simulink model "Tilt_Controller"  (R2016a)
settings: Solver=VariableStepAuto  StartTime=0.0  StopTime=10  FixedStep=Ts  RelTol=1e-3
model workspace (MAT data in the model file):
  AC_ATTITUDE_ACCEL_Y_CONTROLLER_MAX_RADSS = Simulink.Signal
  AC_ATTITUDE_ACCEL_Y_CONTROLLER_MAX_RADSS.DataType = 'double'
  AC_ATTITUDE_ACCEL_Y_CONTROLLER_MAX_RADSS.Dimensions = 1
  AC_ATTITUDE_ACCEL_Y_CONTROLLER_MAX_RADSS.DimensionsMode = 'auto'
  AC_ATTITUDE_ACCEL_Y_CONTROLLER_MAX_RADSS.Complexity = 'real'
  AC_ATTITUDE_ACCEL_Y_CONTROLLER_MAX_RADSS.SampleTime = -1
  AC_ATTITUDE_ACCEL_Y_CONTROLLER_MAX_RADSS.SamplingMode = 'Sample based'
  AC_ATTITUDE_ACCEL_Y_CONTROLLER_MAX_RADSS.InitialValue = '0.5'
  AC_ATTITUDE_CONTROL_MAX = Simulink.Signal
  AC_ATTITUDE_CONTROL_MAX.DataType = 'double'
  AC_ATTITUDE_CONTROL_MAX.Dimensions = 1
  AC_ATTITUDE_CONTROL_MAX.DimensionsMode = 'auto'
  AC_ATTITUDE_CONTROL_MAX.Complexity = 'real'
  AC_ATTITUDE_CONTROL_MAX.SampleTime = -1
  AC_ATTITUDE_CONTROL_MAX.SamplingMode = 'Sample based'
  AC_ATTITUDE_CONTROL_MAX.InitialValue = '0.5'
  AC_ATTITUDE_THRUST_ERROR_ANGLE = Simulink.Signal
  AC_ATTITUDE_THRUST_ERROR_ANGLE.DataType = 'double'
  AC_ATTITUDE_THRUST_ERROR_ANGLE.Dimensions = 1
  AC_ATTITUDE_THRUST_ERROR_ANGLE.DimensionsMode = 'auto'
  AC_ATTITUDE_THRUST_ERROR_ANGLE.Complexity = 'real'
  AC_ATTITUDE_THRUST_ERROR_ANGLE.SampleTime = -1
  AC_ATTITUDE_THRUST_ERROR_ANGLE.SamplingMode = 'Sample based'
  AC_ATTITUDE_THRUST_ERROR_ANGLE.InitialValue = '1000'
  ROLL_PITCH_INPUT_MAX = Simulink.Signal
  ROLL_PITCH_INPUT_MAX.DataType = 'double'
  ROLL_PITCH_INPUT_MAX.Dimensions = 1
  ROLL_PITCH_INPUT_MAX.DimensionsMode = 'auto'
  ROLL_PITCH_INPUT_MAX.Complexity = 'real'
  ROLL_PITCH_INPUT_MAX.SampleTime = -1
  ROLL_PITCH_INPUT_MAX.SamplingMode = 'Sample based'
  ROLL_PITCH_INPUT_MAX.InitialValue = '3000'
  Sig = Simulink.Signal
  Sig.DataType = 'auto'
  Sig.Dimensions = -1
  Sig.DimensionsMode = 'auto'
  Sig.Complexity = 'auto'
  Sig.SampleTime = -1
  Sig.SamplingMode = 'auto'
  Sig1 = Simulink.Signal
  Sig1.DataType = 'auto'
  Sig1.Dimensions = -1
  Sig1.DimensionsMode = 'auto'
  Sig1.Complexity = 'auto'
  Sig1.SampleTime = -1
  Sig1.SamplingMode = 'auto'
  acro_yaw_p = Simulink.Signal
  acro_yaw_p.DataType = 'double'
  acro_yaw_p.Dimensions = 1
  acro_yaw_p.DimensionsMode = 'auto'
  acro_yaw_p.Complexity = 'real'
  acro_yaw_p.SampleTime = -1
  acro_yaw_p.SamplingMode = 'Sample based'
  acro_yaw_p.InitialValue = '45'
  angle_max = Simulink.Signal
  angle_max.DataType = 'double'
  angle_max.Dimensions = 1
  angle_max.DimensionsMode = 'auto'
  angle_max.Complexity = 'real'
  angle_max.SampleTime = -1
  angle_max.SamplingMode = 'Sample based'
  angle_max.InitialValue = '3000'
  attitude_target_ang_vel = Simulink.Signal
  attitude_target_ang_vel.DataType = 'double'
  attitude_target_ang_vel.Dimensions = 3
  attitude_target_ang_vel.DimensionsMode = 'auto'
  attitude_target_ang_vel.Complexity = 'real'
  attitude_target_ang_vel.SampleTime = -1
  attitude_target_ang_vel.SamplingMode = 'Sample based'
  attitude_target_ang_vel.InitialValue = '[0 0 0]'
  attitude_target_euler_angle_x = Simulink.Signal
  attitude_target_euler_angle_x.DataType = 'double'
  attitude_target_euler_angle_x.Dimensions = 1
  attitude_target_euler_angle_x.DimensionsMode = 'auto'
  attitude_target_euler_angle_x.Complexity = 'real'
  attitude_target_euler_angle_x.SampleTime = -1
  attitude_target_euler_angle_x.SamplingMode = 'Sample based'
  attitude_target_euler_angle_x.InitialValue = '0'
  attitude_target_euler_angle_y = Simulink.Signal
  attitude_target_euler_angle_y.DataType = 'double'
  attitude_target_euler_angle_y.Dimensions = 1
  attitude_target_euler_angle_y.DimensionsMode = 'auto'
  attitude_target_euler_angle_y.Complexity = 'real'
  attitude_target_euler_angle_y.SampleTime = -1
  attitude_target_euler_angle_y.SamplingMode = 'Sample based'
  attitude_target_euler_angle_y.InitialValue = '0'
  attitude_target_euler_angle_z = Simulink.Signal
  attitude_target_euler_angle_z.DataType = 'double'
  attitude_target_euler_angle_z.Dimensions = 1
  attitude_target_euler_angle_z.DimensionsMode = 'auto'
  attitude_target_euler_angle_z.Complexity = 'real'
  attitude_target_euler_angle_z.SampleTime = -1
  attitude_target_euler_angle_z.SamplingMode = 'Sample based'
  attitude_target_euler_angle_z.InitialValue = '0'
  attitude_target_euler_rate = Simulink.Signal
  attitude_target_euler_rate.DataType = 'double'
  attitude_target_euler_rate.Dimensions = 3
  attitude_target_euler_rate.DimensionsMode = 'auto'
  attitude_target_euler_rate.Complexity = 'real'
  attitude_target_euler_rate.SampleTime = -1
  attitude_target_euler_rate.SamplingMode = 'Sample based'
  attitude_target_euler_rate.InitialValue = '[0 0 0]'
  attitude_target_quat = Simulink.Signal
  attitude_target_quat.DataType = 'double'
  attitude_target_quat.Dimensions = 4
  attitude_target_quat.DimensionsMode = 'auto'
  attitude_target_quat.Complexity = 'real'
  attitude_target_quat.SampleTime = -1
  attitude_target_quat.SamplingMode = 'Sample based'
  attitude_target_quat.InitialValue = '[1 0 0 0]'
  attitude_vehicle_quat = Simulink.Signal
  attitude_vehicle_quat.DataType = 'double'
  attitude_vehicle_quat.Dimensions = 4
  attitude_vehicle_quat.DimensionsMode = 'auto'
  attitude_vehicle_quat.Complexity = 'real'
  attitude_vehicle_quat.SampleTime = -1
  attitude_vehicle_quat.SamplingMode = 'Sample based'
  attitude_vehicle_quat.InitialValue = '[1 0 0 0]'
  dt = Simulink.Signal
  dt.DataType = 'double'
  dt.Dimensions = 1
  dt.DimensionsMode = 'auto'
  dt.Complexity = 'real'
  dt.SampleTime = -1
  dt.SamplingMode = 'Sample based'
  dt.InitialValue = '0.01'
  false = 0
  limit_roll_pitch = Simulink.Signal
  limit_roll_pitch.DataType = 'double'
  limit_roll_pitch.Dimensions = 1
  limit_roll_pitch.DimensionsMode = 'auto'
  limit_roll_pitch.Complexity = 'real'
  limit_roll_pitch.SampleTime = -1
  limit_roll_pitch.SamplingMode = 'Sample based'
  limit_roll_pitch.InitialValue = '0.0'
  limit_throttle_upper = Simulink.Signal
  limit_throttle_upper.DataType = 'logical'
  limit_throttle_upper.Dimensions = 1
  limit_throttle_upper.DimensionsMode = 'auto'
  limit_throttle_upper.Complexity = 'real'
  limit_throttle_upper.SampleTime = -1
  limit_throttle_upper.SamplingMode = 'Sample based'
  limit_throttle_upper.InitialValue = '0'
  limit_yaw = Simulink.Signal
  limit_yaw.DataType = 'double'
  limit_yaw.Dimensions = 1
  limit_yaw.DimensionsMode = 'auto'
  limit_yaw.Complexity = 'real'
  limit_yaw.SampleTime = -1
  limit_yaw.SamplingMode = 'Sample based'
  limit_yaw.InitialValue = '0'
  loop_rate = Simulink.Signal
  loop_rate.DataType = 'double'
  loop_rate.Dimensions = 1
  loop_rate.DimensionsMode = 'auto'
  loop_rate.Complexity = 'real'
  loop_rate.SampleTime = -1
  loop_rate.SamplingMode = 'Sample based'
  loop_rate.InitialValue = '100'
  pitch_attitude_kP = Simulink.Signal
  pitch_attitude_kP.DataType = 'double'
  pitch_attitude_kP.Dimensions = 1
  pitch_attitude_kP.DimensionsMode = 'auto'
  pitch_attitude_kP.Complexity = 'real'
  pitch_attitude_kP.SampleTime = -1
  pitch_attitude_kP.SamplingMode = 'Sample based'
  pitch_attitude_kP.InitialValue = '20'
  pitch_factor = Simulink.Signal
  pitch_factor.DataType = 'double'
  pitch_factor.Dimensions = 4
  pitch_factor.DimensionsMode = 'auto'
  pitch_factor.Complexity = 'real'
  pitch_factor.SampleTime = -1
  pitch_factor.SamplingMode = 'Sample based'
  pitch_factor.InitialValue = '[cos(deg2rad(15)) -cos(deg2rad(15)) cos(deg2rad(15)) -cos(deg2rad(15))]'
  pitch_rate_derivative = Simulink.Signal
  pitch_rate_derivative.DataType = 'double'
  pitch_rate_derivative.Dimensions = 1
  pitch_rate_derivative.DimensionsMode = 'auto'
  pitch_rate_derivative.Complexity = 'real'
  pitch_rate_derivative.SampleTime = -1
  pitch_rate_derivative.SamplingMode = 'Sample based'
  pitch_rate_derivative.InitialValue = '0'
  pitch_rate_error_rads = Simulink.Signal
  pitch_rate_error_rads.DataType = 'double'
  pitch_rate_error_rads.Dimensions = 1
  pitch_rate_error_rads.DimensionsMode = 'auto'
  pitch_rate_error_rads.Complexity = 'real'
  pitch_rate_error_rads.SampleTime = -1
  pitch_rate_error_rads.SamplingMode = 'Sample based'
  pitch_rate_error_rads.InitialValue = '0'
  pitch_rate_filt_hz = Simulink.Signal
  pitch_rate_filt_hz.DataType = 'double'
  pitch_rate_filt_hz.Dimensions = 1
  pitch_rate_filt_hz.DimensionsMode = 'auto'
  pitch_rate_filt_hz.Complexity = 'real'
  pitch_rate_filt_hz.SampleTime = -1
  pitch_rate_filt_hz.SamplingMode = 'Sample based'
  pitch_rate_filt_hz.InitialValue = '1/(2*pi)'
  pitch_rate_imax = Simulink.Signal
  pitch_rate_imax.DataType = 'double'
  pitch_rate_imax.Dimensions = 1
  pitch_rate_imax.DimensionsMode = 'auto'
  pitch_rate_imax.Complexity = 'real'
  pitch_rate_imax.SampleTime = -1
  pitch_rate_imax.SamplingMode = 'Sample based'
  pitch_rate_imax.InitialValue = '200'
  pitch_rate_integrator = Simulink.Signal
  pitch_rate_integrator.DataType = 'double'
  pitch_rate_integrator.Dimensions = 1
  pitch_rate_integrator.DimensionsMode = 'auto'
  pitch_rate_integrator.Complexity = 'real'
  pitch_rate_integrator.SampleTime = -1
  pitch_rate_integrator.SamplingMode = 'Sample based'
  pitch_rate_integrator.InitialValue = '0'
  pitch_rate_kD = Simulink.Signal
  pitch_rate_kD.DataType = 'double'
  pitch_rate_kD.Dimensions = 1
  pitch_rate_kD.DimensionsMode = 'auto'
  pitch_rate_kD.Complexity = 'real'
  pitch_rate_kD.SampleTime = -1
  pitch_rate_kD.SamplingMode = 'Sample based'
  pitch_rate_kD.InitialValue = '0.004'
  pitch_rate_kI = Simulink.Signal
  pitch_rate_kI.DataType = 'double'
  pitch_rate_kI.Dimensions = 1
  pitch_rate_kI.DimensionsMode = 'auto'
  pitch_rate_kI.Complexity = 'real'
  pitch_rate_kI.SampleTime = -1
  pitch_rate_kI.SamplingMode = 'Sample based'
  pitch_rate_kI.InitialValue = '0.1'
  pitch_rate_kP = Simulink.Signal
  pitch_rate_kP.DataType = 'double'
  pitch_rate_kP.Dimensions = 1
  pitch_rate_kP.DimensionsMode = 'auto'
  pitch_rate_kP.Complexity = 'real'
  pitch_rate_kP.SampleTime = -1
  pitch_rate_kP.SamplingMode = 'Sample based'
  pitch_rate_kP.InitialValue = '0.5'
  pitch_rate_last_input = Simulink.Signal
  pitch_rate_last_input.DataType = 'double'
  pitch_rate_last_input.Dimensions = 1
  pitch_rate_last_input.DimensionsMode = 'auto'
  pitch_rate_last_input.Complexity = 'real'
  pitch_rate_last_input.SampleTime = -1
  pitch_rate_last_input.SamplingMode = 'Sample based'
  pitch_rate_last_input.InitialValue = '0'
  pitch_rate_proportional = Simulink.Signal
  pitch_rate_proportional.DataType = 'double'
  pitch_rate_proportional.Dimensions = 1
  pitch_rate_proportional.DimensionsMode = 'auto'
  pitch_rate_proportional.Complexity = 'real'
  pitch_rate_proportional.SampleTime = -1
  pitch_rate_proportional.SamplingMode = 'Sample based'
  pitch_rate_proportional.InitialValue = '0'
  pwm_max = Simulink.Signal
  pwm_max.DataType = 'double'
  pwm_max.Dimensions = 1
  pwm_max.DimensionsMode = 'auto'
  pwm_max.Complexity = 'real'
  pwm_max.SampleTime = -1
  pwm_max.SamplingMode = 'Sample based'
  pwm_max.InitialValue = '2000'
  pwm_min = Simulink.Signal
  pwm_min.DataType = 'double'
  pwm_min.Dimensions = 1
  pwm_min.DimensionsMode = 'auto'
  pwm_min.Complexity = 'real'
  pwm_min.SampleTime = -1
  pwm_min.SamplingMode = 'Sample based'
  pwm_min.InitialValue = '1039'
  rate_bf_ff_enabled = Simulink.Signal
  rate_bf_ff_enabled.DataType = 'double'
  rate_bf_ff_enabled.Dimensions = 1
  rate_bf_ff_enabled.DimensionsMode = 'auto'
  rate_bf_ff_enabled.Complexity = 'real'
  rate_bf_ff_enabled.SampleTime = -1
  rate_bf_ff_enabled.SamplingMode = 'Sample based'
  rate_bf_ff_enabled.InitialValue = '0'
  rate_target_ang_vel = Simulink.Signal
  rate_target_ang_vel.DataType = 'double'
  rate_target_ang_vel.Dimensions = 3
  rate_target_ang_vel.DimensionsMode = 'auto'
  rate_target_ang_vel.Complexity = 'real'
  rate_target_ang_vel.SampleTime = -1
  rate_target_ang_vel.SamplingMode = 'Sample based'
  rate_target_ang_vel.InitialValue = '[0 0 0]'
  roll_attitude_kP = Simulink.Signal
  roll_attitude_kP.DataType = 'double'
  roll_attitude_kP.Dimensions = 1
  roll_attitude_kP.DimensionsMode = 'auto'
  roll_attitude_kP.Complexity = 'real'
  roll_attitude_kP.SampleTime = -1
  roll_attitude_kP.SamplingMode = 'Sample based'
  roll_attitude_kP.InitialValue = '20'
  roll_factor = Simulink.Signal
  roll_factor.DataType = 'double'
  roll_factor.Dimensions = 4
  roll_factor.DimensionsMode = 'auto'
  roll_factor.Complexity = 'real'
  roll_factor.SampleTime = -1
  roll_factor.SamplingMode = 'Sample based'
  roll_factor.InitialValue = '[-sin(deg2rad(15)) sin(deg2rad(15)) sin(deg2rad(15)) -sin(deg2rad(15))]'
  roll_rate_derivative = Simulink.Signal
  roll_rate_derivative.DataType = 'double'
  roll_rate_derivative.Dimensions = 1
  roll_rate_derivative.DimensionsMode = 'auto'
  roll_rate_derivative.Complexity = 'real'
  roll_rate_derivative.SampleTime = -1
  roll_rate_derivative.SamplingMode = 'Sample based'
  roll_rate_derivative.InitialValue = '0'
  roll_rate_error_rads = Simulink.Signal
  roll_rate_error_rads.DataType = 'double'
  roll_rate_error_rads.Dimensions = 1
  roll_rate_error_rads.DimensionsMode = 'auto'
  roll_rate_error_rads.Complexity = 'real'
  roll_rate_error_rads.SampleTime = -1
  roll_rate_error_rads.SamplingMode = 'Sample based'
  roll_rate_error_rads.InitialValue = '0'
  roll_rate_filt_hz = Simulink.Signal
  roll_rate_filt_hz.DataType = 'double'
  roll_rate_filt_hz.Dimensions = 1
  roll_rate_filt_hz.DimensionsMode = 'auto'
  roll_rate_filt_hz.Complexity = 'real'
  roll_rate_filt_hz.SampleTime = -1
  roll_rate_filt_hz.SamplingMode = 'Sample based'
  roll_rate_filt_hz.InitialValue = '1/(2*pi)'
  roll_rate_imax = Simulink.Signal
  roll_rate_imax.DataType = 'double'
  roll_rate_imax.Dimensions = 1
  roll_rate_imax.DimensionsMode = 'auto'
  roll_rate_imax.Complexity = 'real'
  roll_rate_imax.SampleTime = -1
  roll_rate_imax.SamplingMode = 'Sample based'
  roll_rate_imax.InitialValue = '200'
  roll_rate_integrator = Simulink.Signal
  roll_rate_integrator.DataType = 'double'
  roll_rate_integrator.Dimensions = 1
  roll_rate_integrator.DimensionsMode = 'auto'
  roll_rate_integrator.Complexity = 'real'
  roll_rate_integrator.SampleTime = -1
  roll_rate_integrator.SamplingMode = 'Sample based'
  roll_rate_integrator.InitialValue = '0'
  roll_rate_kD = Simulink.Signal
  roll_rate_kD.DataType = 'double'
  roll_rate_kD.Dimensions = 1
  roll_rate_kD.DimensionsMode = 'auto'
  roll_rate_kD.Complexity = 'real'
  roll_rate_kD.SampleTime = -1
  roll_rate_kD.SamplingMode = 'Sample based'
  roll_rate_kD.InitialValue = '0.004'
  roll_rate_kI = Simulink.Signal
  roll_rate_kI.DataType = 'double'
  roll_rate_kI.Dimensions = 1
  roll_rate_kI.DimensionsMode = 'auto'
  roll_rate_kI.Complexity = 'real'
  roll_rate_kI.SampleTime = -1
  roll_rate_kI.SamplingMode = 'Sample based'
  roll_rate_kI.InitialValue = '0.1'
  roll_rate_kP = Simulink.Signal
  roll_rate_kP.DataType = 'double'
  roll_rate_kP.Dimensions = 1
  roll_rate_kP.DimensionsMode = 'auto'
  roll_rate_kP.Complexity = 'real'
  roll_rate_kP.SampleTime = -1
  roll_rate_kP.SamplingMode = 'Sample based'
  roll_rate_kP.InitialValue = '1'
  roll_rate_last_input = Simulink.Signal
  roll_rate_last_input.DataType = 'double'
  roll_rate_last_input.Dimensions = 1
  roll_rate_last_input.DimensionsMode = 'auto'
  roll_rate_last_input.Complexity = 'real'
  roll_rate_last_input.SampleTime = -1
  roll_rate_last_input.SamplingMode = 'Sample based'
  roll_rate_last_input.InitialValue = '0'
  roll_rate_proportional = Simulink.Signal
  roll_rate_proportional.DataType = 'double'
  roll_rate_proportional.Dimensions = 1
  roll_rate_proportional.DimensionsMode = 'auto'
  roll_rate_proportional.Complexity = 'real'
  roll_rate_proportional.SampleTime = -1
  roll_rate_proportional.SamplingMode = 'Sample based'
  roll_rate_proportional.InitialValue = '0'
  spin_max = Simulink.Signal
  spin_max.DataType = 'double'
  spin_max.Dimensions = 1
  spin_max.DimensionsMode = 'auto'
  spin_max.Complexity = 'real'
  spin_max.SampleTime = -1
  spin_max.SamplingMode = 'Sample based'
  spin_max.InitialValue = '0.95'
  spin_min = Simulink.Signal
  spin_min.DataType = 'double'
  spin_min.Dimensions = 1
  spin_min.DimensionsMode = 'auto'
  spin_min.Complexity = 'real'
  spin_min.SampleTime = -1
  spin_min.SamplingMode = 'Sample based'
  spin_min.InitialValue = '0.15'
  throttle_avg_max = Simulink.Signal
  throttle_avg_max.DataType = 'double'
  throttle_avg_max.Dimensions = 1
  throttle_avg_max.DimensionsMode = 'auto'
  throttle_avg_max.Complexity = 'real'
  throttle_avg_max.SampleTime = -1
  throttle_avg_max.SamplingMode = 'Sample based'
  throttle_avg_max.InitialValue = '0'
  throttle_filter_cutoff_freq = Simulink.Signal
  throttle_filter_cutoff_freq.DataType = 'double'
  throttle_filter_cutoff_freq.Dimensions = 1
  throttle_filter_cutoff_freq.DimensionsMode = 'auto'
  throttle_filter_cutoff_freq.Complexity = 'real'
  throttle_filter_cutoff_freq.SampleTime = -1
  throttle_filter_cutoff_freq.SamplingMode = 'Sample based'
  throttle_filter_cutoff_freq.InitialValue = '0.5'
  throttle_filter_output = Simulink.Signal
  throttle_filter_output.DataType = 'double'
  throttle_filter_output.Dimensions = 1
  throttle_filter_output.DimensionsMode = 'auto'
  throttle_filter_output.Complexity = 'real'
  throttle_filter_output.SampleTime = -1
  throttle_filter_output.SamplingMode = 'Sample based'
  throttle_filter_output.InitialValue = '0'
  throttle_in = Simulink.Signal
  throttle_in.DataType = 'double'
  throttle_in.Dimensions = 1
  throttle_in.DimensionsMode = 'auto'
  throttle_in.Complexity = 'real'
  throttle_in.SampleTime = -1
  throttle_in.SamplingMode = 'Sample based'
  throttle_in.InitialValue = '0'
  throttle_rpy_mix = Simulink.Signal
  throttle_rpy_mix.DataType = 'double'
  throttle_rpy_mix.Dimensions = 1
  throttle_rpy_mix.DimensionsMode = 'auto'
  throttle_rpy_mix.Complexity = 'real'
  throttle_rpy_mix.SampleTime = -1
  throttle_rpy_mix.SamplingMode = 'Sample based'
  throttle_rpy_mix.InitialValue = '0'
  throttle_rpy_mix_desired = Simulink.Signal
  throttle_rpy_mix_desired.DataType = 'double'
  throttle_rpy_mix_desired.Dimensions = 1
  throttle_rpy_mix_desired.DimensionsMode = 'auto'
  throttle_rpy_mix_desired.Complexity = 'real'
  throttle_rpy_mix_desired.SampleTime = -1
  throttle_rpy_mix_desired.SamplingMode = 'Sample based'
  throttle_rpy_mix_desired.InitialValue = '0'
  throttle_thrust = Simulink.Signal
  throttle_thrust.DataType = 'double'
  throttle_thrust.Dimensions = 1
  throttle_thrust.DimensionsMode = 'auto'
  throttle_thrust.Complexity = 'real'
  throttle_thrust.SampleTime = -1
  throttle_thrust.SamplingMode = 'Sample based'
  throttle_thrust.InitialValue = '0'
  throttle_thrust_best_rpy = Simulink.Signal
  throttle_thrust_best_rpy.DataType = 'double'
  throttle_thrust_best_rpy.Dimensions = 1
  throttle_thrust_best_rpy.DimensionsMode = 'auto'
  throttle_thrust_best_rpy.Complexity = 'real'
  throttle_thrust_best_rpy.SampleTime = -1
  throttle_thrust_best_rpy.SamplingMode = 'Sample based'
  throttle_thrust_best_rpy.InitialValue = '0'
  throttle_thrust_max = Simulink.Signal
  throttle_thrust_max.DataType = 'double'
  throttle_thrust_max.Dimensions = 1
  throttle_thrust_max.DimensionsMode = 'auto'
  throttle_thrust_max.Complexity = 'real'
  throttle_thrust_max.SampleTime = -1
  throttle_thrust_max.SamplingMode = 'Sample based'
  throttle_thrust_max.InitialValue = '1'
  thrust_error_angle = Simulink.Signal
  thrust_error_angle.DataType = 'double'
  thrust_error_angle.Dimensions = 1
  thrust_error_angle.DimensionsMode = 'auto'
  thrust_error_angle.Complexity = 'real'
  thrust_error_angle.SampleTime = -1
  thrust_error_angle.SamplingMode = 'Sample based'
  thrust_error_angle.InitialValue = '0'
  thrust_rpyt_out = Simulink.Signal
  thrust_rpyt_out.DataType = 'double'
  thrust_rpyt_out.Dimensions = 4
  thrust_rpyt_out.DimensionsMode = 'auto'
  thrust_rpyt_out.Complexity = 'real'
  thrust_rpyt_out.SampleTime = -1
  thrust_rpyt_out.SamplingMode = 'Sample based'
  thrust_rpyt_out.InitialValue = '[0 0 0 0]'
  true = 1
  use_ff_and_input_shaping = Simulink.Signal
  use_ff_and_input_shaping.DataType = 'double'
  use_ff_and_input_shaping.Dimensions = 1
  use_ff_and_input_shaping.DimensionsMode = 'auto'
  use_ff_and_input_shaping.Complexity = 'real'
  use_ff_and_input_shaping.SampleTime = -1
  use_ff_and_input_shaping.SamplingMode = 'Sample based'
  use_ff_and_input_shaping.InitialValue = '0'
  variableType = 'S'
  yaw_allowed = Simulink.Signal
  yaw_allowed.DataType = 'double'
  yaw_allowed.Dimensions = 1
  yaw_allowed.DimensionsMode = 'auto'
  yaw_allowed.Complexity = 'real'
  yaw_allowed.SampleTime = -1
  yaw_allowed.SamplingMode = 'Sample based'
  yaw_allowed.InitialValue = '1'
  yaw_attitude_kP = Simulink.Signal
  yaw_attitude_kP.DataType = 'double'
  yaw_attitude_kP.Dimensions = 1
  yaw_attitude_kP.DimensionsMode = 'auto'
  yaw_attitude_kP.Complexity = 'real'
  yaw_attitude_kP.SampleTime = -1
  yaw_attitude_kP.SamplingMode = 'Sample based'
  yaw_attitude_kP.InitialValue = '4.5'
  yaw_factor = Simulink.Signal
  yaw_factor.DataType = 'double'
  yaw_factor.Dimensions = 4
  yaw_factor.DimensionsMode = 'auto'
  yaw_factor.Complexity = 'real'
  yaw_factor.SampleTime = -1
  yaw_factor.SamplingMode = 'Sample based'
  yaw_factor.InitialValue = '[0.1 0.1 -0.1 -0.1]'
  yaw_headroom = Simulink.Signal
  yaw_headroom.DataType = 'double'
  yaw_headroom.Dimensions = 1
  yaw_headroom.DimensionsMode = 'auto'
  yaw_headroom.Complexity = 'real'
  yaw_headroom.SampleTime = -1
  yaw_headroom.SamplingMode = 'Sample based'
  yaw_headroom.InitialValue = '200'
  yaw_rate_derivative = Simulink.Signal
  yaw_rate_derivative.DataType = 'double'
  yaw_rate_derivative.Dimensions = 1
  yaw_rate_derivative.DimensionsMode = 'auto'
  yaw_rate_derivative.Complexity = 'real'
  yaw_rate_derivative.SampleTime = -1
  yaw_rate_derivative.SamplingMode = 'Sample based'
  yaw_rate_derivative.InitialValue = '0'
  yaw_rate_error_rads = Simulink.Signal
  yaw_rate_error_rads.DataType = 'double'
  yaw_rate_error_rads.Dimensions = 1
  yaw_rate_error_rads.DimensionsMode = 'auto'
  yaw_rate_error_rads.Complexity = 'real'
  yaw_rate_error_rads.SampleTime = -1
  yaw_rate_error_rads.SamplingMode = 'Sample based'
  yaw_rate_error_rads.InitialValue = '0'
  yaw_rate_filt_hz = Simulink.Signal
  yaw_rate_filt_hz.DataType = 'double'
  yaw_rate_filt_hz.Dimensions = 1
  yaw_rate_filt_hz.DimensionsMode = 'auto'
  yaw_rate_filt_hz.Complexity = 'real'
  yaw_rate_filt_hz.SampleTime = -1
  yaw_rate_filt_hz.SamplingMode = 'Sample based'
  yaw_rate_filt_hz.InitialValue = '1/(2*pi)'
  yaw_rate_imax = Simulink.Signal
  yaw_rate_imax.DataType = 'double'
  yaw_rate_imax.Dimensions = 1
  yaw_rate_imax.DimensionsMode = 'auto'
  yaw_rate_imax.Complexity = 'real'
  yaw_rate_imax.SampleTime = -1
  yaw_rate_imax.SamplingMode = 'Sample based'
  yaw_rate_imax.InitialValue = '200'
  yaw_rate_integrator = Simulink.Signal
  yaw_rate_integrator.DataType = 'double'
  yaw_rate_integrator.Dimensions = 1
  yaw_rate_integrator.DimensionsMode = 'auto'
  yaw_rate_integrator.Complexity = 'real'
  yaw_rate_integrator.SampleTime = -1
  yaw_rate_integrator.SamplingMode = 'Sample based'
  yaw_rate_integrator.InitialValue = '0'
  yaw_rate_kD = Simulink.Signal
  yaw_rate_kD.DataType = 'double'
  yaw_rate_kD.Dimensions = 1
  yaw_rate_kD.DimensionsMode = 'auto'
  yaw_rate_kD.Complexity = 'real'
  yaw_rate_kD.SampleTime = -1
  yaw_rate_kD.SamplingMode = 'Sample based'
  yaw_rate_kD.InitialValue = '5'
  yaw_rate_kI = Simulink.Signal
  yaw_rate_kI.DataType = 'double'
  yaw_rate_kI.Dimensions = 1
  yaw_rate_kI.DimensionsMode = 'auto'
  yaw_rate_kI.Complexity = 'real'
  yaw_rate_kI.SampleTime = -1
  yaw_rate_kI.SamplingMode = 'Sample based'
  yaw_rate_kI.InitialValue = '0.1'
  yaw_rate_kP = Simulink.Signal
  yaw_rate_kP.DataType = 'double'
  yaw_rate_kP.Dimensions = 1
  yaw_rate_kP.DimensionsMode = 'auto'
  yaw_rate_kP.Complexity = 'real'
  yaw_rate_kP.SampleTime = -1
  yaw_rate_kP.SamplingMode = 'Sample based'
  yaw_rate_kP.InitialValue = '0.2'
  yaw_rate_last_input = Simulink.Signal
  yaw_rate_last_input.DataType = 'double'
  yaw_rate_last_input.Dimensions = 1
  yaw_rate_last_input.DimensionsMode = 'auto'
  yaw_rate_last_input.Complexity = 'real'
  yaw_rate_last_input.SampleTime = -1
  yaw_rate_last_input.SamplingMode = 'Sample based'
  yaw_rate_last_input.InitialValue = '0'
  yaw_rate_proportional = Simulink.Signal
  yaw_rate_proportional.DataType = 'double'
  yaw_rate_proportional.Dimensions = 1
  yaw_rate_proportional.DimensionsMode = 'auto'
  yaw_rate_proportional.Complexity = 'real'
  yaw_rate_proportional.SampleTime = -1
  yaw_rate_proportional.SamplingMode = 'Sample based'
  yaw_rate_proportional.InitialValue = '0'
libraries: simulink_extras x6, vrlib x2, aerolibtransform2 x2, aerolibutil x1
settings Model: Creator=s121814  LastModifiedBy=GusBus
settings SolverCC: ZeroCrossControl=DisableAll
settings DataIOCC: SaveFormat=Array  SaveState=on

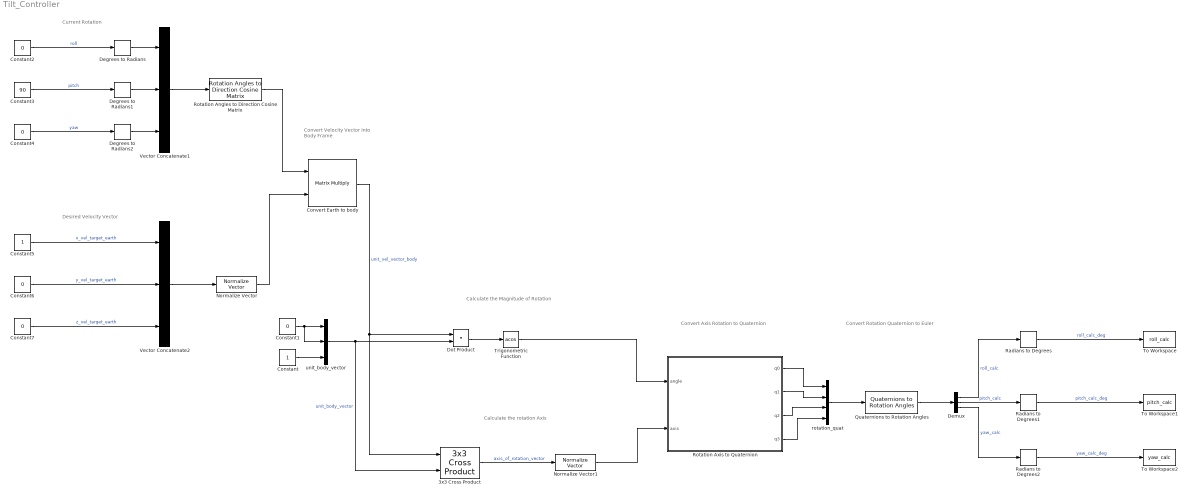
== system Tilt_Controller ==
  note: Convert Rotation Quaternion to Euler
  note: Convert Axis Rotation to Quaternion
  note: Calculate the rotation Axis
  note: Desired Velocity Vector
  note: Current Rotation
  note: Convert Velocity Vector into Body Frame
  note: Calculate the Magnitude of Rotation
  3x3 Cross Product : aerolibutil/3x3 Cross Product
  Constant : Constant
  Constant{1..2,4,6..7} (5 alike) : Constant  Value=0
  Constant3 : Constant  Value=90
  Constant5 : Constant
  Convert Earth to body : Product  Multiplication=Matrix(*)
  Degrees to Radians : simulink_extras/Transformations/Degrees to Radians
  Degrees to Radians1 : simulink_extras/Transformations/Degrees to Radians
  Degrees to Radians2 : simulink_extras/Transformations/Degrees to Radians
  Demux : Demux  Outputs=3
  Dot Product : DotProduct  InputSameDT=on  OutDataTypeStr=Inherit: Inherit via internal rule
  Normalize Vector : vrlib/Utilities/Normalize Vector  maxzero=0
  Normalize Vector1 : vrlib/Utilities/Normalize Vector  maxzero=0
  Quaternions to Rotation Angles : aerolibtransform2/Quaternions to Rotation Angles  rotationOrder=XYZ
  Radians to Degrees : simulink_extras/Transformations/Radians to Degrees
  Radians to Degrees1 : simulink_extras/Transformations/Radians to Degrees
  Radians to Degrees2 : simulink_extras/Transformations/Radians to Degrees
  Rotation Angles to Direction Cosine Matrix : aerolibtransform2/Rotation Angles to Direction Cosine Matrix  rotationOrder=XYZ
  Rotation Axis to Quaternion : MATLAB Function  TreatAsAtomicUnit=on
  To Workspace : ToWorkspace  VariableName=roll_calc  SaveFormat=Timeseries  SampleTime=-1
  To Workspace1 : ToWorkspace  VariableName=pitch_calc  SaveFormat=Timeseries  SampleTime=-1
  To Workspace2 : ToWorkspace  VariableName=yaw_calc  SaveFormat=Timeseries  SampleTime=-1
  Trigonometric Function : Trigonometry  Operator=acos
  Vector Concatenate1 : Concatenate  NumInputs=3
  Vector Concatenate2 : Concatenate  NumInputs=3
  rotation_quat : Concatenate  NumInputs=4
  unit_body_vector : Concatenate  NumInputs=3
  wires:
  Constant5/1 -> Vector Concatenate2/1  "x_vel_target_earth"
  Constant6/1 -> Vector Concatenate2/2  "y_vel_target_earth"
  Constant7/1 -> Vector Concatenate2/3  "z_vel_target_earth"
  Vector Concatenate2/1 -> Normalize Vector/1
  Convert Earth to body/1 -> Dot Product/1, 3x3 Cross Product/1  "unit_vel_vector_body"
  Constant1/1 -> unit_body_vector/2, unit_body_vector/1
  Constant/1 -> unit_body_vector/3
  unit_body_vector/1 -> Dot Product/2, 3x3 Cross Product/2  "unit_body_vector"
  3x3 Cross Product/1 -> Normalize Vector1/1  "axis_of_rotation_vector"
  Normalize Vector/1 -> Convert Earth to body/2
  Dot Product/1 -> Trigonometric Function/1
  Trigonometric Function/1 -> Rotation Axis to Quaternion/1(angle)
  Normalize Vector1/1 -> Rotation Axis to Quaternion/2(axis)
  Quaternions to Rotation Angles/1 -> Demux/1
  Demux/1 -> Radians to Degrees/1  "roll_calc"
  Demux/2 -> Radians to Degrees1/1  "pitch_calc"
  Demux/3 -> Radians to Degrees2/1  "yaw_calc"
  rotation_quat/1 -> Quaternions to Rotation Angles/1
  Rotation Angles to Direction Cosine Matrix/1 -> Convert Earth to body/1
  Constant2/1 -> Degrees to Radians/1  "roll"
  Constant3/1 -> Degrees to Radians1/1  "pitch"
  Constant4/1 -> Degrees to Radians2/1  "yaw"
  Vector Concatenate1/1 -> Rotation Angles to Direction Cosine Matrix/1
  Degrees to Radians/1 -> Vector Concatenate1/1
  Degrees to Radians1/1 -> Vector Concatenate1/2
  Degrees to Radians2/1 -> Vector Concatenate1/3
  Rotation Axis to Quaternion/1(q0) -> rotation_quat/1
  Rotation Axis to Quaternion/2(q1) -> rotation_quat/2
  Rotation Axis to Quaternion/3(q2) -> rotation_quat/3
  Rotation Axis to Quaternion/4(q3) -> rotation_quat/4
  Radians to Degrees/1 -> To Workspace/1  "roll_calc_deg"
  Radians to Degrees1/1 -> To Workspace1/1  "pitch_calc_deg"
  Radians to Degrees2/1 -> To Workspace2/1  "yaw_calc_deg"

== matlab function Tilt_Controller/Rotation Axis to Quaternion ==
  data: q0 output; angle input; q1 output; axis input; q2 output; q3 output
function [q0, q1, q2, q3]= rotation_axis_to_quaternion(angle, axis)
%#codegen

q0 = cos(angle/2);
q1 = axis(1) * sin(angle/2);
q2 = axis(2) * sin(angle/2);
q3 = axis(3) * sin(angle/2);
% q3 = 0;


% http://www.euclideanspace.com/maths/geometry/rotations/conversions/angleToQuaternion/index.htm
% http://www.euclideanspace.com/maths/geometry/rotations/conversions/angleToQuaternion/examples/index.htm
